simulink model "lab4teleia3"  (R2021a)
settings: Solver=ode23tb  StartTime=0.0  StopTime=30  MaxStep=1e-5  RelTol=1e-3
libraries: spsRMSLib x1, simulink x1, spsSynchronousMachineSIFundamentalLib x1, spspowerguiLib x1
settings Model: Creator=sotos  LastModifiedBy=sotos

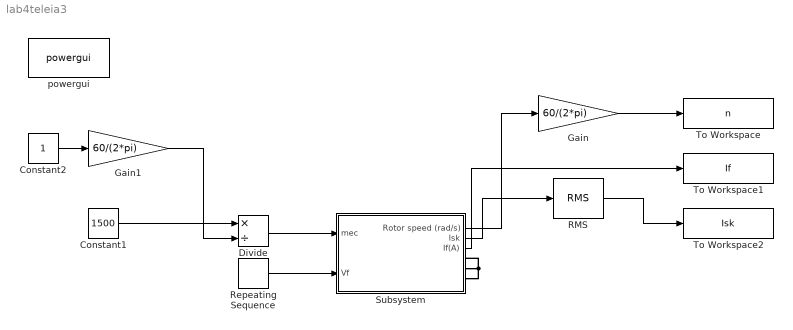
== system lab4teleia3 ==
  Constant1 : Constant  Value=1500
  Constant2 : Constant
  Divide : Product  Inputs=*/
  Gain : Gain  Gain=60/(2*pi)
  Gain1 : Gain  Gain=60/(2*pi)
  RMS : spsRMSLib/RMS  TrueRMS=on  Freq=50  RMSInit=0  Ts=0
  Repeating Sequence : simulink/Sources/Repeating Sequence  rep_seq_t=t  rep_seq_y=V
  Subsystem : Subsystem
      mask DialogControl Label1 Prompt: 8.1kVA, 400V, 4 poles
  To Workspace : ToWorkspace  VariableName=n  SaveFormat=Timeseries  SampleTime=-1
  To Workspace1 : ToWorkspace  VariableName=If  SaveFormat=Timeseries  SampleTime=-1
  To Workspace2 : ToWorkspace  VariableName=Isk  SaveFormat=Timeseries  SampleTime=-1
  powergui : spspowerguiLib/powergui  Priority=1  SimulationMode=Continuous  SampleTime=50e-6  frequency=60  Iterations=50  frequencyindice=50  Pbase=100e6  ErrMax=1e-4  UnitsV=kV  UnitsW=MW  buscounter=0  FunctionMessages=off  echomessages=off  EnableUseOfTLC=off  CurrentSourceSwitches=off  DisableSnubberDevices=off  DisableRonSwitches=off  DisableVfSwitches=off  DisplayEquations=off  AutomaticDiscreteSolvers=off  SolverType=Tustin/Backward Euler (TBE)  Interpol=off  ExternalGateDelay=off  methode=off  Ts=100  x0status=blocks  SPID=on  SwTol=0  HookPort=off  NonlinearTolerance=1e-4  nMaxIteration=100  ContinueOnMaxIteration=off  RestoreLinks=warning  ResistiveCurrentMeasurement=off  Frange=[0:2:500]  Ylog=off  Xlog=on  ShowGrid=off  save=off  variable=ZData  structure=0  ZoomFFT=off  StartTime=0.0  cycles=1  DisplayStyle=1  fundamental=60  FreqAxis=off  MaxFrequency=1000  frequencyindicesteady=1  RmsSteady=1  display=off
  wires:
  Subsystem/1(Rotor speed (rad/s)) -> Gain/1
  Subsystem/2(Isk) -> RMS/1
  RMS/1 -> To Workspace2/1
  Subsystem/3(Ιf(A)) -> To Workspace1/1
  Gain/1 -> To Workspace/1
  Divide/1 -> Subsystem/1(mec)
  Repeating Sequence/1 -> Subsystem/2(Vf)
  Constant1/1 -> Divide/1
  Gain1/1 -> Divide/2
  Constant2/1 -> Gain1/1
  connections:
  Subsystem/RConn3 -- Subsystem/RConn1 -- Subsystem/RConn2

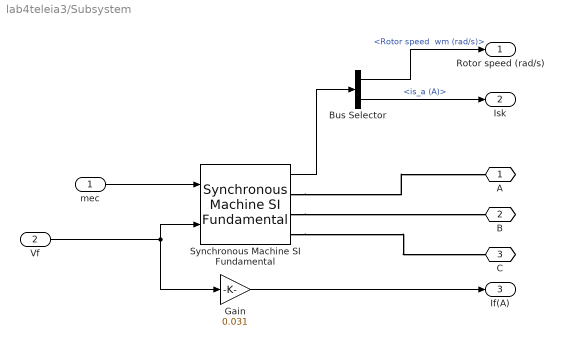
== system lab4teleia3/Subsystem ==
  mec : Inport
  Vf : Inport  Port=2
  Bus Selector : BusSelector  OutputSignals="Mechanical.Rotor speed  wm (rad/s),Stator current.is_a (A)"
  Gain : Gain  Gain=0.031
  Synchronous Machine SI Fundamental : spsSynchronousMachineSIFundamentalLib/Synchronous Machine SI Fundamental  PresetModel=No  MechanicalLoad=Speed w  ShowDetailedParameters=on  RotorType=Salient-pole  Units=SI fundamental parameters  MeasurementBus=off  NominalParameters=[8100 400 50 7]  Stator=[1.62 0.004527 0.1086 0.05175]  Field=[1.208 0.01132]  Dampers2=[ 0.0664, 1.387e-3, 0.0292, 6.896e-4, 7.907e-3, 2.477e-3]  Dampers1=[3.142 0.007334 4.772 0.01015]  Mechanical=[0.0923 0.009 2]  PolePairs=2  InitialConditions="[ 0  0  0  0  0  0  0  0  1]"  SetSaturation=on  Saturation=[695.64,774.7,917.5,1001.6,1082.2,1175.9,1293.6,1430.2,1583.7;9660,10623,12243,13063,13757,14437,15180,15890,16567]  DisplayVfd=off  LoadFlowParameters=[1,0,0,0,0]  TsPowergui=0  TsBlock=-1  IterativeModel=Trapezoidal non iterative  IterativeDiscreteModel=Trapezoidal non iterative  BusType=PV  Pref=0  Qref=0  Qmin=-inf  Qmax=inf  PLF=0  QLF=0
      settings: SourceProductBaseCode=PS
  A : PMIOPort  Side=Right
  B : PMIOPort  Port=2  Side=Right
  C : PMIOPort  Port=3  Side=Right
  Rotor speed (rad/s) : Outport
  Isk : Outport  Port=2
  Ιf(A) : Outport  Port=3
  wires:
  Synchronous Machine SI Fundamental/1 -> Bus Selector/1
  mec/1 -> Synchronous Machine SI Fundamental/1
  Bus Selector/1 -> Rotor speed (rad/s)/1  "<Rotor speed  wm (rad/s)>"
  Vf/1 -> Gain/1, Synchronous Machine SI Fundamental/2
  Gain/1 -> Ιf(A)/1
  Bus Selector/2 -> Isk/1  "<is_a (A)>"
  connections:
  Synchronous Machine SI Fundamental/RConn2 -- B/RConn1
  Synchronous Machine SI Fundamental/RConn1 -- A/RConn1
  Synchronous Machine SI Fundamental/RConn3 -- C/RConn1
